simulink model "Oil"  (Simulink 7.9)
settings: Solver=VariableStepDiscrete  StartTime=0.0  StopTime=8  RelTol=1e-3
libraries: slident x2
settings Model: Creator=Saeed  LastModifiedBy=Saeed

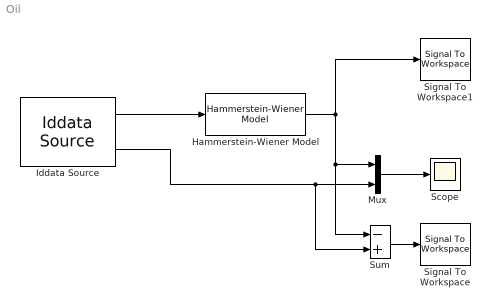
== system Oil ==
  Hammerstein-Wiener Model : slident/Hammerstein-Wiener Model  sys=CO1  IC=State values  X0i=x0
  Iddata Source : slident/Iddata Source  iddataobj=XX
  Mux : Mux  Inputs=2
  Scope : Scope
  Signal To Workspace : SignalToWorkspace  VariableName=yout
      settings: CopyFcn=dspblkcopystw(gcbh);
  Signal To Workspace1 : SignalToWorkspace  VariableName=mout
      settings: CopyFcn=dspblkcopystw(gcbh);
  Sum : Sum  Inputs=-+
  wires:
  Iddata Source/1 -> Hammerstein-Wiener Model/1
  Hammerstein-Wiener Model/1 -> Signal To Workspace1/1, Mux/1, Sum/1
  Mux/1 -> Scope/1
  Iddata Source/2 -> Mux/2, Sum/2
  Sum/1 -> Signal To Workspace/1
